simulink model "Simulation"  (R2017b)
settings: Solver=VariableStepAuto  StartTime=0.0  StopTime=3  RelTol=1e-3
settings Model: Creator=Aloysio  LastModifiedBy=aloysio
settings CodeAppCC: StateflowObjectComments=on
settings SimscapeCC: SimscapeNormalizeSystem=off

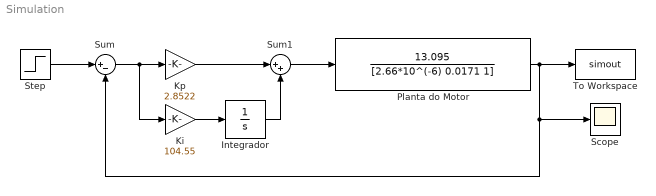
== system Simulation ==
  Integrador : TransferFcn  Denominator=[1 0]
  Ki : Gain  Gain=104.55
  Kp : Gain  Gain=2.8522
  Planta do Motor : TransferFcn  Numerator=[13.095]  Denominator=[2.66*10^(-6) 0.0171 1]
  Scope : Scope
  Step : Step  After=100  SampleTime=0
  Sum : Sum  Inputs=|+-
  Sum1 : Sum  Inputs=|++
  To Workspace : ToWorkspace  VariableName=simout  SaveFormat=Timeseries  SampleTime=-1
  wires:
  Planta do Motor/1 -> Sum/2, Scope/1, To Workspace/1
  Step/1 -> Sum/1
  Sum1/1 -> Planta do Motor/1
  Ki/1 -> Integrador/1
  Kp/1 -> Sum1/1
  Integrador/1 -> Sum1/2
  Sum/1 -> Ki/1, Kp/1
